simulink model "serial_plot_v1"  (R2019a)
settings: Solver=VariableStepAuto  StartTime=0.0  StopTime=inf  RelTol=1e-3
libraries: instrumentlib x2
settings Model: Creator=facuolmed_o  LastModifiedBy=facuolmed_o

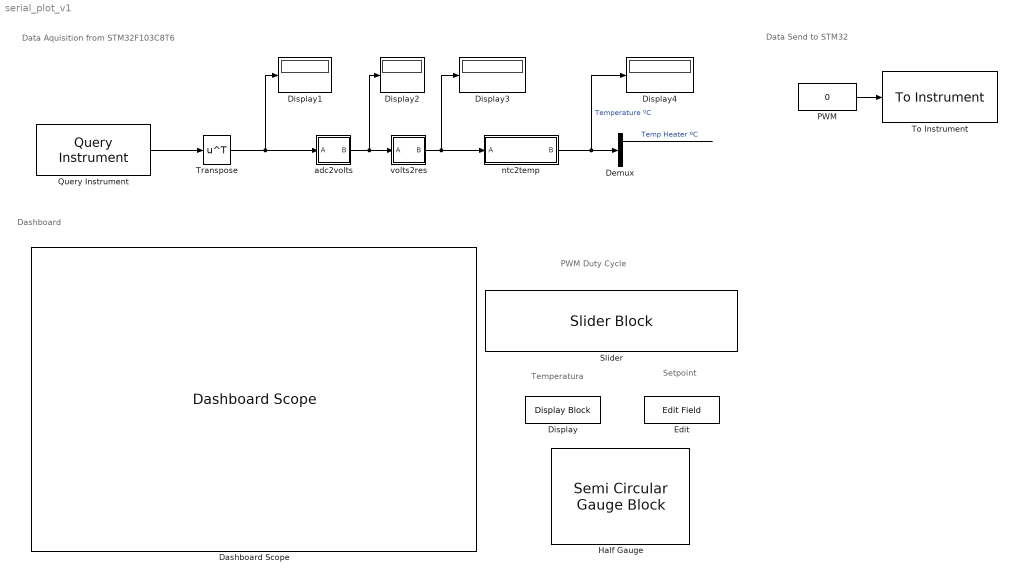
== system serial_plot_v1 ==
  note: PWM Duty Cycle
  note: Data Send to STM32
  note: Dashboard
  note: Data Aquisition from STM32F103C8T6
  note: Temperatura
  note: Setpoint
  Dashboard Scope : DashboardScope  TimeSpan=1000  Ymax=400  ScaleAtStop=off
  Demux : Demux  Outputs=2
  Display : DisplayBlock  LabelPosition=Hide  Format=short
  Display{1..4} (4 alike) : Display
      settings: Format=bank
  Edit : EditField  LabelPosition=Hide  ShowInitialText=on  Alignment=Center
  Half Gauge : SemiCircularGaugeBlock  ScaleMax=400
  "PWM " : Constant  Value=0  OutDataTypeStr=double  SampleTime=0
  Query Instrument : instrumentlib/Query Instrument  sampleTime=0  isWorkspaceObject=off  timeout=10  inputBufferSize=512  protocol=Serial  serialPort=COM2  baudRate=115200  gpibVendor=Keysight Technologies  boardIndex=0  primaryAddress=1  secondaryAddress=0  visaVendor=Keysight  visaSerialPort=0  chassisIndex=0  logicalAddress=0  tcpRemoteHost='127.0.0.1'  tcpRemotePort=4500  udpRemoteHost='127.0.0.1'  udpRemotePort=9090  visaTCPBoardIndex=0  visaTCPRemoteHost='127.0.0.1'  usbBoardIndex=0  usbManufID=0  usbModelCode=0  usbSerialNumber=0  initAction=None  initCommand='DATA:SOURCE CH1'  initFunction=get  queryCommand=''  responseFormat=ASCII  asciiFormatting='%d,%d\n'  precision=8-bit unsigned integer  byteOrder=Little endian  valuesToRead=1  removeBytes=off  afterOutputAction=Repeat query for new data  enableFrames=on  frameSize=2
      settings: SourceProductName=Instrument Control Toolbox  SourceProductBaseCode=IC
  Slider : SliderBlock  ScaleMax=255
  To Instrument : instrumentlib/To Instrument  sampleTime=0  isWorkspaceObject=off  timeout=10  inputBufferSize=100  protocol=Serial  serialPort=COM2  baudRate=115200  gpibVendor=ICS Electronics  boardIndex=0  primaryAddress=1  secondaryAddress=0  visaVendor=Keysight  visaSerialPort=0  chassisIndex=0  logicalAddress=0  tcpRemoteHost='127.0.0.1'  tcpRemotePort=4500  udpRemoteHost='127.0.0.1'  udpRemotePort=9090  visaTCPBoardIndex=0  visaTCPRemoteHost='127.0.0.1'  usbBoardIndex=0  usbManufID=0  usbModelCode=0  usbSerialNumber=0  initAction=None  initCommand='DATA:SOURCE CH1'  initFunction=get  command=''  sendFormat=Binary  asciiFormatting='%c'  precision=8-bit unsigned integer  byteOrder=Little endian
      settings: SourceProductName=Instrument Control Toolbox  SourceProductBaseCode=IC
  Transpose : Math  Operator=transpose  SaturateOnIntegerOverflow=on
  adc2volts : Subsystem
  ntc2temp : Subsystem
  volts2res : Subsystem
  wires:
  Query Instrument/1 -> Transpose/1
  Transpose/1 -> Display1/1, adc2volts/1(A)
  "PWM "/1 -> To Instrument/1
  adc2volts/1(B) -> volts2res/1(A), Display2/1
  volts2res/1(B) -> ntc2temp/1(A), Display3/1
  ntc2temp/1(B) -> Demux/1, Display4/1  "Temperature ºC"
  Demux/1 -> ?  "Temp Heater ºC"

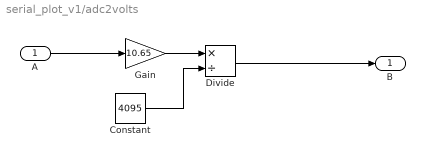
== system serial_plot_v1/adc2volts ==
  A : Inport
  Constant : Constant  Value=4095
  Divide : Product  Inputs=*/
  Gain : Gain  Gain=10.65
  B : Outport
  wires:
  A/1 -> Gain/1
  Gain/1 -> Divide/1
  Divide/1 -> B/1
  Constant/1 -> Divide/2

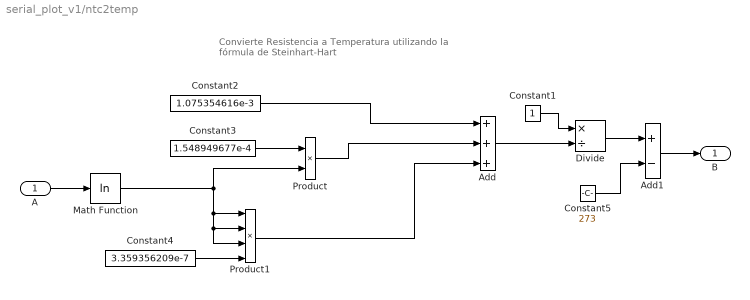
== system serial_plot_v1/ntc2temp ==
  note: Convierte Resistencia a Temperatura utilizando la fórmula de Steinhart-Hart
  A : Inport
  Add : Sum  Inputs=+++
  Add1 : Sum  Inputs=+-
  Constant1 : Constant
  Constant2 : Constant  Value=1.075354616e-3
  Constant3 : Constant  Value=1.548949677e-4
  Constant4 : Constant  Value=3.359356209e-7
  Constant5 : Constant  Value=273
  Divide : Product  Inputs=*/
  Math Function : Math  Operator=log  SaturateOnIntegerOverflow=on
  Product : Product
  Product1 : Product  Inputs=4
  B : Outport
  wires:
  Constant1/1 -> Divide/1
  A/1 -> Math Function/1
  Constant2/1 -> Add/1
  Constant3/1 -> Product/1
  Math Function/1 -> Product1/3, Product1/2, Product1/1, Product/2
  Product/1 -> Add/2
  Add/1 -> Divide/2
  Constant4/1 -> Product1/4
  Product1/1 -> Add/3
  Divide/1 -> Add1/1
  Constant5/1 -> Add1/2
  Add1/1 -> B/1

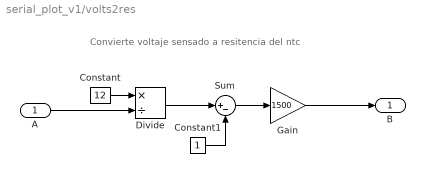
== system serial_plot_v1/volts2res ==
  note: Convierte voltaje sensado a resitencia del ntc
  A : Inport
  Constant : Constant  Value=12
  Constant1 : Constant
  Divide : Product  Inputs=*/
  Gain : Gain  Gain=1500
  Sum : Sum  Inputs=|+-
  B : Outport
  wires:
  Constant/1 -> Divide/1
  A/1 -> Divide/2
  Divide/1 -> Sum/1
  Constant1/1 -> Sum/2
  Sum/1 -> Gain/1
  Gain/1 -> B/1
